simulink model "testbed"  (R2024a)
settings: Solver=ode4  StartTime=0.0  StopTime=300  FixedStep=0.1  RelTol=1e-3
libraries: simulink x2, rllib x1, slpidlib x1
settings Model: Creator=Vasilis  LastModifiedBy=Vassilis

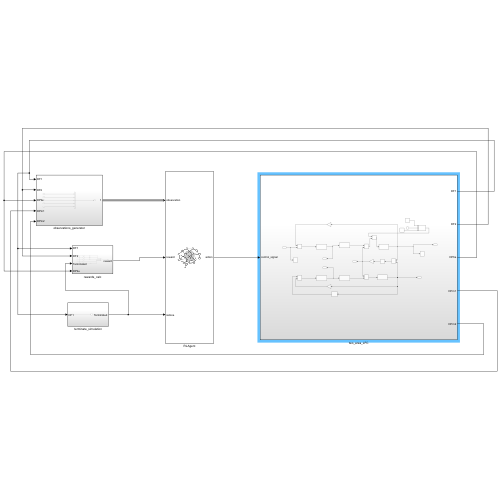
[thumbnail: Simulink's stored preview of the top-level diagram]
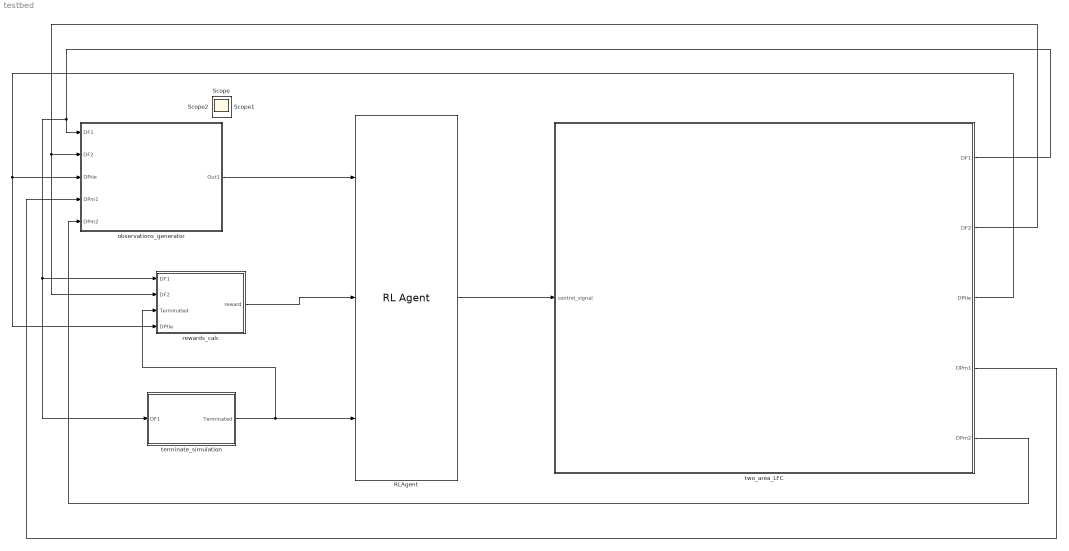
== system testbed ==
  RLAgent : rllib/RL Agent  Agent=agentObj  ExternalActionAsInput=off  ProvideLastAction=off  ProvideCumRwd=off  TreatAsDirectFeedthrough=on  UseStrictObservationDataTypes=off
  observations_generator : Subsystem
  rewards_calc : Subsystem
  terminate_simulation : Subsystem
  two_area_LFC : Subsystem
  Scope : Scope
  Scope1 : Scope
  Scope2 : Scope
  wires:
  observations_generator/1(Out1) -> RLAgent/1
  two_area_LFC/1(DF1) -> rewards_calc/1(DF1), terminate_simulation/1(DF1), observations_generator/1(DF1)
  two_area_LFC/2(DF2) -> rewards_calc/2(DF2), observations_generator/2(DF2)
  two_area_LFC/3(DPtie) -> rewards_calc/4(DPtie), observations_generator/3(DPtie)
  two_area_LFC/4(DPm1) -> observations_generator/4(DPm1)
  two_area_LFC/5(DPm2) -> observations_generator/5(DPm2)
  RLAgent/1 -> two_area_LFC/1(control_signal)
  terminate_simulation/1(Terminated) -> rewards_calc/3(Terminated), RLAgent/3
  rewards_calc/1(reward) -> RLAgent/2

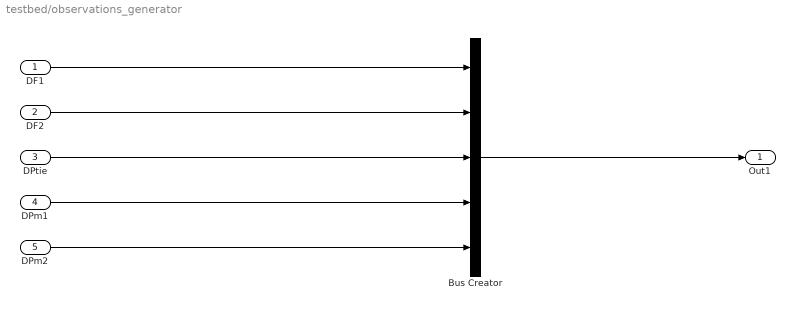
== system testbed/observations_generator ==
  DF1 : Inport
  DF2 : Inport  Port=2
  DPtie : Inport  Port=3
  DPm1 : Inport  Port=4
  DPm2 : Inport  Port=5
  Bus Creator : BusCreator  Inputs=5
  Out1 : Outport
  wires:
  Bus Creator/1 -> Out1/1
  DF1/1 -> Bus Creator/1
  DF2/1 -> Bus Creator/2
  DPtie/1 -> Bus Creator/3
  DPm1/1 -> Bus Creator/4
  DPm2/1 -> Bus Creator/5

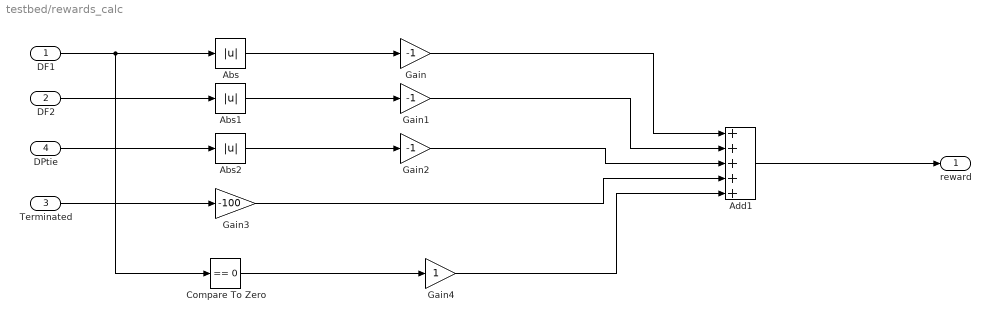
== system testbed/rewards_calc ==
  DF1 : Inport
  DF2 : Inport  Port=2
  Terminated : Inport  Port=3
  DPtie : Inport  Port=4
  Abs : Abs  SaturateOnIntegerOverflow=off
  Abs1 : Abs  SaturateOnIntegerOverflow=off
  Abs2 : Abs  SaturateOnIntegerOverflow=off
  Add1 : Sum  Inputs=+++++
  Compare To Zero : simulink/Logic and Bit Operations/Compare To Zero  relop===  OutDataTypeStr=boolean
  Gain : Gain  Gain=-1
  Gain1 : Gain  Gain=-1
  Gain2 : Gain  Gain=-1
  Gain3 : Gain  Gain=-100
  Gain4 : Gain
  reward : Outport
  wires:
  Gain1/1 -> Add1/2
  Abs/1 -> Gain/1
  Abs2/1 -> Gain2/1
  Gain/1 -> Add1/1
  Gain3/1 -> Add1/4
  Terminated/1 -> Gain3/1
  Compare To Zero/1 -> Gain4/1
  DPtie/1 -> Abs2/1
  Abs1/1 -> Gain1/1
  Gain4/1 -> Add1/5
  DF1/1 -> Compare To Zero/1, Abs/1
  DF2/1 -> Abs1/1
  Gain2/1 -> Add1/3
  Add1/1 -> reward/1

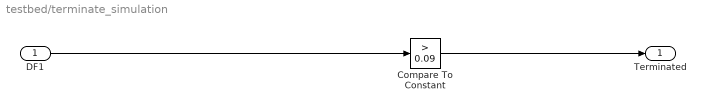
== system testbed/terminate_simulation ==
  DF1 : Inport
  Compare To Constant : simulink/Logic and Bit Operations/Compare To Constant  relop=>  const=0.09  OutDataTypeStr=boolean
  Terminated : Outport
  wires:
  DF1/1 -> Compare To Constant/1
  Compare To Constant/1 -> Terminated/1

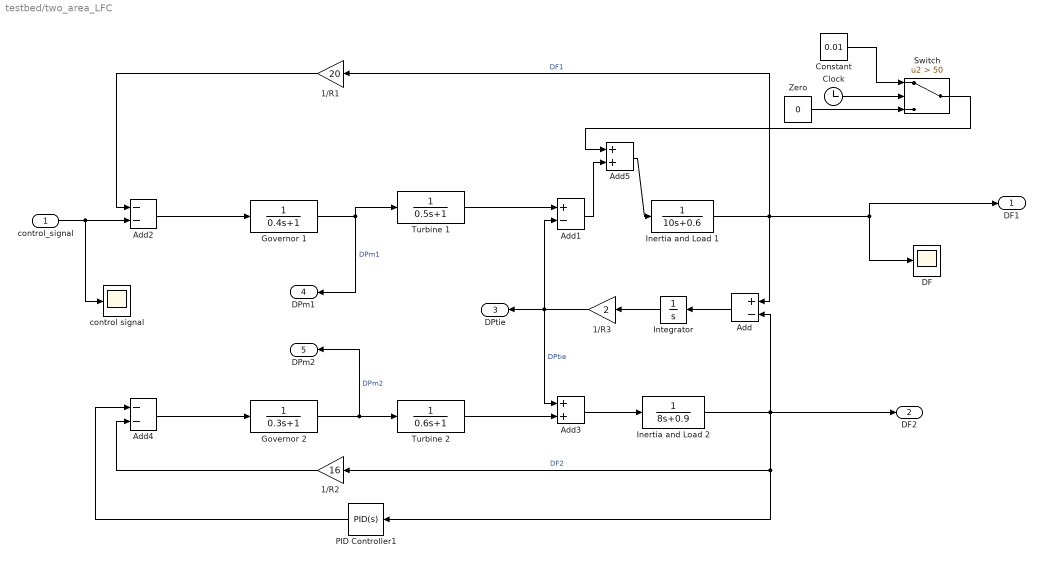
== system testbed/two_area_LFC ==
  control_signal : Inport  OutMin=[-0.005]  OutMax=[0.005]
  " Turbine 1" : TransferFcn  Denominator=[0.5 1]
  " Turbine 2" : TransferFcn  Denominator=[0.6 1]
  1/R1 : Gain  Gain=20
  1/R2 : Gain  Gain=16
  1/R3 : Gain  Gain=2
  Add : Sum  Inputs=+-
  Add1 : Sum  Inputs=+-
  Add2 : Sum  Inputs=--
  Add3 : Sum
  Add4 : Sum  Inputs=--
  Add5 : Sum
  Clock : Clock
  Constant : Constant  Value=0.01
  DF : Scope
  Governor 1 : TransferFcn  Denominator=[0.4 1]
  Governor 2 : TransferFcn  Denominator=[0.3 1]
  Inertia and Load 1 : TransferFcn  Denominator=[10 0.6]
  Inertia and Load 2 : TransferFcn  Denominator=[8 0.9]
  Integrator : Integrator
  PID Controller1 : slpidlib/PID Controller  Controller=PID  Form=Parallel  TimeDomain=Continuous-time  UseExternalTs=off  SampleTime=-1  IntegratorMethod=Forward Euler  FilterMethod=Forward Euler  ControllerParametersSource=internal  P=1  I=1  UseKiTs=off  D=0  UseExternalDerivativeSource=off  N=100  UseFilter=on  TunerSelectOption=Transfer Function Based (PID Tuner App)  InitialConditionSource=internal  InitialConditionForIntegrator=0  InitialConditionForFilter=0  DifferentiatorICPrevScaledInput=0  ExternalReset=none  TrackingMode=off  Kt=1  LimitOutput=off  SatLimitsSource=internal  UpperSaturationLimit=inf  LowerSaturationLimit=-inf  LinearizeAsGain=on  AntiWindupMode=none  Kb=1  LimitIntegrator=off  UpperIntegratorSaturationLimit=inf  LowerIntegratorSaturationLimit=-inf  POutMin=[]  POutMax=[]  IOutMin=[]  IOutMax=[]  DOutMin=[]  DOutMax=[]  NOutMin=[]  NOutMax=[]  SumOutMin=[]  SumOutMax=[]  SaturationOutMin=[]  SaturationOutMax=[]  PParamMin=[]  PParamMax=[]  IParamMin=[]  IParamMax=[]  DParamMin=[]  DParamMax=[]  NParamMin=[]  NParamMax=[]  KbParamMin=[]  KbParamMax=[]  KtParamMin=[]  KtParamMax=[]  KbOutMin=[]  KbOutMax=[]  KtOutMin=[]  KtOutMax=[]  IntegratorOutMin=[]  IntegratorOutMax=[]  FilterOutMin=[]  FilterOutMax=[]  SumI1OutMin=[]  SumI1OutMax=[]  SumI2OutMin=[]  SumI2OutMax=[]  SumI3OutMin=[]  SumI3OutMax=[]  SumI4OutMin=[]  SumI4OutMax=[]  SumDOutMin=[]  SumDOutMax=[]  DifferentiatorOutMin=[]  DifferentiatorOutMax=[]  FilterDiffOutCoefMin=[]  FilterDiffOutCoefMax=[]  ReciprocalOutMin=[]  ReciprocalOutMax=[]  SumDenOutMin=[]  SumDenOutMax=[]  SumNumOutMin=[]  SumNumOutMax=[]  DivideOutMin=[]  DivideOutMax=[]  UdiffTsProdOutMin=[]  UdiffTsProdOutMax=[]  NTsProdOutMin=[]  NTsProdOutMax=[]  UintegralTsProdOutMin=[]  UintegralTsProdOutMax=[]  UngainTsProdOutMin=[]  UngainTsProdOutMax=[]  ClampingZeroOutDataTypeStr=Inherit: Inherit via back propagation  ClampingZeroOutMin=[]  ClampingZeroOutMax=[]  FilterDenConstantOutDataTypeStr=Inherit: Inherit via back propagation  FilterDenConstantOutMin=[]  FilterDenConstantOutMax=[]  PCopyOutDataTypeStr=Inherit: Inherit via back propagation  PCopyOutMin=[]  PCopyOutMax=[]  NCopyOutDataTypeStr=Inherit: Inherit via back propagation  NCopyOutMin=[]  NCopyOutMax=[]  IntegratorContinuousStateAttributes=''  IntegratorStateMustResolveToSignalObject=off  IntegratorRTWStateStorageClass=Auto  FilterContinuousStateAttributes=''  FilterStateMustResolveToSignalObject=off  FilterRTWStateStorageClass=Auto  ParallelPVariant=InternalParameters  IdealPVariant=Disabled  IVariant=InternalParameters  DVariant=InternalParameters  IntegratorVariant=Continuous  SatVariant=Disabled  AWVariant=Passthrough  PCopyVariant=Disabled  TRVariant=Disabled  FdbkBlocksVariant=Forward  IdealPFdbkVariant=Disabled  SatFdbkVariant=Disabled  DerivativeFilterVariant=ContFilter  NVariant=InternalParameters  NCopyVariant=Disabled  FilterICVariant=InternalICsFilter  IntegratorICVariant=InternalICs  ExternalResetVariant=Disabled  TRSumVariant=Passthrough  SumFdbkVariant=Disabled  SumVariant=Sum_PID  TsampFilterVariant=InternalTs  TsampNgainVariant=Passthrough  TsampIntegralVariant=Disabled_SignalSpec  ExternalSaturationOutDataTypeStr=Inherit: Same as second input  DerivativeSourceVariant=ErrorSignal
  Switch : Switch  Criteria=u2 > Threshold  Threshold=50  SaturateOnIntegerOverflow=off  InputSameDT=off
  Zero : Constant  Value=0  OutDataTypeStr=Inherit: Inherit via back propagation
  control signal : Scope
  DF1 : Outport
  DF2 : Outport  Port=2
  DPtie : Outport  Port=3
  DPm1 : Outport  Port=4
  DPm2 : Outport  Port=5
  wires:
  Inertia and Load 2/1 -> Add/2, DF2/1, PID Controller1/1, 1/R2/1  "DF2"
  Inertia and Load 1/1 -> Add/1, DF/1, DF1/1, 1/R1/1  "DF1"
  Add4/1 -> Governor 2/1
  Add3/1 -> Inertia and Load 2/1
  " Turbine 1"/1 -> Add1/1
  1/R1/1 -> Add2/1
  Governor 2/1 -> DPm2/1, " Turbine 2"/1  "DPm2"
  " Turbine 2"/1 -> Add3/2
  Add/1 -> Integrator/1
  1/R2/1 -> Add4/2
  Governor 1/1 -> DPm1/1, " Turbine 1"/1  "DPm1"
  Add2/1 -> Governor 1/1
  PID Controller1/1 -> Add4/1
  Integrator/1 -> 1/R3/1
  1/R3/1 -> Add3/1, DPtie/1, Add1/2  "DPtie"
  control_signal/1 -> Add2/2, control signal/1
  Clock/1 -> Switch/2
  Zero/1 -> Switch/3
  Add1/1 -> Add5/2
  Add5/1 -> Inertia and Load 1/1
  Switch/1 -> Add5/1
  Constant/1 -> Switch/1
